simulink model "FRNmodel"  (Simulink 7.9)
settings: Solver=VariableStepDiscrete  StartTime=0.0  StopTime=100.0  RelTol=1e-3
libraries: simeventslib x22, FRN_Library x11
(part 2 of 2)

== system FRNmodel/LTL/Calculate_OUTFlow ==
  Calculate_OUTFlow : MATLAB Function  TreatAsAtomicUnit=on
  Entity Combiner : EntityCombiner  NumberInputPorts=2
  Entity Sink : EntitySink
  Entity Splitter : EntitySplitter  NumberOutputPorts=2
  FIFO Queue : FIFOQueue  Capacity=inf
  Get Attribute : GetAttribute  AttributeName=UoH|Quantity|OUTFlow  AttributeMissing=Error|Error|Error  AttributeDefaultValue=1|1|1  AttributeTreatAsVector=1|1|1  AttributeSendTiming=After entity departure|After entity departure|After entity departure  EvaluatedDefaultAttributeValue={[];[];[]}
      settings: OutputPortMap=o1,o2,o3
  Set Attribute : SetAttribute  AttributeName=OUTFlow  AttributeFrom=Signal port  EvaluatedAttributeValue={[]}
  Single Server : SingleServer  ServiceTime=0
  FlowRecord_IN : PMIOPort  Port=1  Side=Left
  FlowRecord_OUT : PMIOPort  Port=2  Side=Left
  OUTFlow_Signal : PMIOPort  Port=3  Side=Right
  wires:
  Get Attribute/3 -> Calculate_OUTFlow/3(OUTFlow)
  Get Attribute/2 -> Calculate_OUTFlow/2(Quantity)
  Calculate_OUTFlow/1(OUTFlow_return) -> Set Attribute/1
  Get Attribute/1 -> Calculate_OUTFlow/1(UoH)
  connections:
  Entity Splitter/RConn2 -- Entity Sink/LConn1
  FIFO Queue/RConn1 -- Entity Combiner/LConn2
  OUTFlow_Signal/RConn1 -- FIFO Queue/LConn1
  FlowRecord_IN/RConn1 -- Entity Combiner/LConn1
  FlowRecord_OUT/RConn1 -- Entity Splitter/RConn1
  Single Server/RConn1 -- Set Attribute/LConn1
  Get Attribute/RConn1 -- Single Server/LConn1
  Set Attribute/RConn1 -- Entity Splitter/LConn1
  Entity Combiner/RConn1 -- Get Attribute/LConn1

== system FRNmodel/LTL/FlowRecord ==
  FIFO Queue : FIFOQueue
  FlowRecord : TimeBasedFunctionCallGenerator  EventGenerationMode=Only at simulation start
  Get Attribute : GetAttribute  AttributeName=OUTFlow|INFlow  AttributeMissing=Error|Error  AttributeDefaultValue=1|1  AttributeTreatAsVector=1|1  AttributeSendTiming=After entity departure|After entity departure  EvaluatedDefaultAttributeValue={[];[]}
      settings: OutputPortMap=o1,o2
  INFlow_Metric : simeventslib/SimEvents Sinks/Discrete Event Signal to Workspace  VariableName=INFlow_Metric_LTL  SaveFormat=Structure With Time  isMonitorOnly=off  isRecordIC=off
  Initialize_FlowRecord : SetAttribute  AttributeName=INFlow|OUTFlow  AttributeFrom=Dialog|Dialog  AttributeValue=[0 0 0 0 0]|[0 0 0 0 0]  AttributeTreatAsVector=1|1  EvaluatedAttributeValue={[0 0 0 0 0];[0 0 0 0 0]}
  New_FlowRecord : EventBasedEntityGenerator  GenerateEntitiesUpon=Function call from port fcn
  OUTFlow_Metric : simeventslib/SimEvents Sinks/Discrete Event Signal to Workspace  VariableName=OUTFlow_Metric_LTL  SaveFormat=Structure With Time  isMonitorOnly=off  isRecordIC=off
  Output Switch : OutputSwitch  NumberOutputPorts=2
  Path Combiner1 : PathCombiner
  TO_INFlow : PMIOPort  Port=1  Side=Right
  TO_OUTFlow : PMIOPort  Port=2  Side=Left
  FROM_INFlow : PMIOPort  Port=3  Side=Right
  FROM_OUTFlow : PMIOPort  Port=4  Side=Left
  wires:
  Get Attribute/2 -> INFlow_Metric/1
  Get Attribute/1 -> OUTFlow_Metric/1
  FlowRecord/1 -> New_FlowRecord/1
  connections:
  Get Attribute/RConn1 -- FIFO Queue/LConn1
  Path Combiner1/RConn1 -- Get Attribute/LConn1
  FROM_OUTFlow/RConn1 -- Path Combiner1/LConn3
  FROM_INFlow/RConn1 -- Path Combiner1/LConn2
  TO_OUTFlow/RConn1 -- Output Switch/RConn2
  TO_INFlow/RConn1 -- Output Switch/RConn1
  Initialize_FlowRecord/RConn1 -- Path Combiner1/LConn1
  New_FlowRecord/RConn1 -- Initialize_FlowRecord/LConn1
  Output Switch/LConn1 -- FIFO Queue/RConn1

== system FRNmodel/MixedPallet/Calculate_INFlow ==
  Calculate_INFlow : MATLAB Function  TreatAsAtomicUnit=on
  Entity Combiner : EntityCombiner  NumberInputPorts=2
  Entity Sink : EntitySink
  Entity Splitter : EntitySplitter  NumberOutputPorts=2
  FIFO Queue : FIFOQueue  Capacity=inf
  Get Attribute : GetAttribute  AttributeName=UoH|Quantity|INFlow  AttributeMissing=Error|Error|Error  AttributeDefaultValue=1|1|1  AttributeTreatAsVector=1|1|1  AttributeSendTiming=After entity departure|After entity departure|After entity departure  EvaluatedDefaultAttributeValue={[];[];[]}
      settings: OutputPortMap=o1,o2,o3
  Set Attribute : SetAttribute  AttributeName=INFlow  AttributeFrom=Signal port  EvaluatedAttributeValue={[]}
  Single Server : SingleServer  ServiceTime=0
  FlowRecord_IN : PMIOPort  Port=1  Side=Right
  FlowRecord_OUT : PMIOPort  Port=2  Side=Right
  INFlow_Signal : PMIOPort  Port=3  Side=Left
  wires:
  Get Attribute/3 -> Calculate_INFlow/3(INFlow)
  Get Attribute/2 -> Calculate_INFlow/2(Quantity)
  Calculate_INFlow/1(INFlow_return) -> Set Attribute/1
  Get Attribute/1 -> Calculate_INFlow/1(UoH)
  connections:
  FIFO Queue/RConn1 -- Entity Combiner/LConn2
  INFlow_Signal/RConn1 -- FIFO Queue/LConn1
  Entity Splitter/RConn2 -- Entity Sink/LConn1
  FlowRecord_IN/RConn1 -- Entity Combiner/LConn1
  FlowRecord_OUT/RConn1 -- Entity Splitter/RConn1
  Single Server/RConn1 -- Set Attribute/LConn1
  Get Attribute/RConn1 -- Single Server/LConn1
  Set Attribute/RConn1 -- Entity Splitter/LConn1
  Entity Combiner/RConn1 -- Get Attribute/LConn1

== system FRNmodel/MixedPallet/Calculate_OUTFlow ==
  Calculate_OUTFlow : MATLAB Function  TreatAsAtomicUnit=on
  Entity Combiner : EntityCombiner  NumberInputPorts=2
  Entity Sink : EntitySink
  Entity Splitter : EntitySplitter  NumberOutputPorts=2
  FIFO Queue : FIFOQueue  Capacity=inf
  Get Attribute : GetAttribute  AttributeName=UoH|Quantity|OUTFlow  AttributeMissing=Error|Error|Error  AttributeDefaultValue=1|1|1  AttributeTreatAsVector=1|1|1  AttributeSendTiming=After entity departure|After entity departure|After entity departure  EvaluatedDefaultAttributeValue={[];[];[]}
      settings: OutputPortMap=o1,o2,o3
  Set Attribute : SetAttribute  AttributeName=OUTFlow  AttributeFrom=Signal port  EvaluatedAttributeValue={[]}
  Single Server : SingleServer  ServiceTime=0
  FlowRecord_IN : PMIOPort  Port=1  Side=Left
  FlowRecord_OUT : PMIOPort  Port=2  Side=Left
  OUTFlow_Signal : PMIOPort  Port=3  Side=Right
  wires:
  Get Attribute/3 -> Calculate_OUTFlow/3(OUTFlow)
  Get Attribute/2 -> Calculate_OUTFlow/2(Quantity)
  Calculate_OUTFlow/1(OUTFlow_return) -> Set Attribute/1
  Get Attribute/1 -> Calculate_OUTFlow/1(UoH)
  connections:
  Entity Splitter/RConn2 -- Entity Sink/LConn1
  FIFO Queue/RConn1 -- Entity Combiner/LConn2
  OUTFlow_Signal/RConn1 -- FIFO Queue/LConn1
  FlowRecord_IN/RConn1 -- Entity Combiner/LConn1
  FlowRecord_OUT/RConn1 -- Entity Splitter/RConn1
  Single Server/RConn1 -- Set Attribute/LConn1
  Get Attribute/RConn1 -- Single Server/LConn1
  Set Attribute/RConn1 -- Entity Splitter/LConn1
  Entity Combiner/RConn1 -- Get Attribute/LConn1

== system FRNmodel/MixedPallet/FlowRecord ==
  FIFO Queue : FIFOQueue
  FlowRecord : TimeBasedFunctionCallGenerator  EventGenerationMode=Only at simulation start
  Get Attribute : GetAttribute  AttributeName=OUTFlow|INFlow  AttributeMissing=Error|Error  AttributeDefaultValue=1|1  AttributeTreatAsVector=1|1  AttributeSendTiming=After entity departure|After entity departure  EvaluatedDefaultAttributeValue={[];[]}
      settings: OutputPortMap=o1,o2
  INFlow_Metric : simeventslib/SimEvents Sinks/Discrete Event Signal to Workspace  VariableName=INFlow_Metric_MixedPallet  SaveFormat=Structure With Time  isMonitorOnly=off  isRecordIC=off
  Initialize_FlowRecord : SetAttribute  AttributeName=INFlow|OUTFlow  AttributeFrom=Dialog|Dialog  AttributeValue=[0 0 0 0 0]|[0 0 0 0 0]  AttributeTreatAsVector=1|1  EvaluatedAttributeValue={[0 0 0 0 0];[0 0 0 0 0]}
  New_FlowRecord : EventBasedEntityGenerator  GenerateEntitiesUpon=Function call from port fcn
  OUTFlow_Metric : simeventslib/SimEvents Sinks/Discrete Event Signal to Workspace  VariableName=OUTFlow_Metric_MixedPallet  SaveFormat=Structure With Time  isMonitorOnly=off  isRecordIC=off
  Output Switch : OutputSwitch  NumberOutputPorts=2
  Path Combiner1 : PathCombiner
  TO_INFlow : PMIOPort  Port=1  Side=Right
  TO_OUTFlow : PMIOPort  Port=2  Side=Left
  FROM_INFlow : PMIOPort  Port=3  Side=Right
  FROM_OUTFlow : PMIOPort  Port=4  Side=Left
  wires:
  Get Attribute/2 -> INFlow_Metric/1
  Get Attribute/1 -> OUTFlow_Metric/1
  FlowRecord/1 -> New_FlowRecord/1
  connections:
  Get Attribute/RConn1 -- FIFO Queue/LConn1
  Path Combiner1/RConn1 -- Get Attribute/LConn1
  FROM_OUTFlow/RConn1 -- Path Combiner1/LConn3
  FROM_INFlow/RConn1 -- Path Combiner1/LConn2
  TO_OUTFlow/RConn1 -- Output Switch/RConn2
  TO_INFlow/RConn1 -- Output Switch/RConn1
  Initialize_FlowRecord/RConn1 -- Path Combiner1/LConn1
  New_FlowRecord/RConn1 -- Initialize_FlowRecord/LConn1
  Output Switch/LConn1 -- FIFO Queue/RConn1

== system FRNmodel/PickFastCarton/Calculate_INFlow ==
  Calculate_INFlow : MATLAB Function  TreatAsAtomicUnit=on
  Entity Combiner : EntityCombiner  NumberInputPorts=2
  Entity Sink : EntitySink
  Entity Splitter : EntitySplitter  NumberOutputPorts=2
  FIFO Queue : FIFOQueue  Capacity=inf
  Get Attribute : GetAttribute  AttributeName=UoH|Quantity|INFlow  AttributeMissing=Error|Error|Error  AttributeDefaultValue=1|1|1  AttributeTreatAsVector=1|1|1  AttributeSendTiming=After entity departure|After entity departure|After entity departure  EvaluatedDefaultAttributeValue={[];[];[]}
      settings: OutputPortMap=o1,o2,o3
  Set Attribute : SetAttribute  AttributeName=INFlow  AttributeFrom=Signal port  EvaluatedAttributeValue={[]}
  Single Server : SingleServer  ServiceTime=0
  FlowRecord_IN : PMIOPort  Port=1  Side=Right
  FlowRecord_OUT : PMIOPort  Port=2  Side=Right
  INFlow_Signal : PMIOPort  Port=3  Side=Left
  wires:
  Get Attribute/3 -> Calculate_INFlow/3(INFlow)
  Get Attribute/2 -> Calculate_INFlow/2(Quantity)
  Calculate_INFlow/1(INFlow_return) -> Set Attribute/1
  Get Attribute/1 -> Calculate_INFlow/1(UoH)
  connections:
  FIFO Queue/RConn1 -- Entity Combiner/LConn2
  INFlow_Signal/RConn1 -- FIFO Queue/LConn1
  Entity Splitter/RConn2 -- Entity Sink/LConn1
  FlowRecord_IN/RConn1 -- Entity Combiner/LConn1
  FlowRecord_OUT/RConn1 -- Entity Splitter/RConn1
  Single Server/RConn1 -- Set Attribute/LConn1
  Get Attribute/RConn1 -- Single Server/LConn1
  Set Attribute/RConn1 -- Entity Splitter/LConn1
  Entity Combiner/RConn1 -- Get Attribute/LConn1

== system FRNmodel/PickFastCarton/Calculate_OUTFlow ==
  Calculate_OUTFlow : MATLAB Function  TreatAsAtomicUnit=on
  Entity Combiner : EntityCombiner  NumberInputPorts=2
  Entity Sink : EntitySink
  Entity Splitter : EntitySplitter  NumberOutputPorts=2
  FIFO Queue : FIFOQueue  Capacity=inf
  Get Attribute : GetAttribute  AttributeName=UoH|Quantity|OUTFlow  AttributeMissing=Error|Error|Error  AttributeDefaultValue=1|1|1  AttributeTreatAsVector=1|1|1  AttributeSendTiming=After entity departure|After entity departure|After entity departure  EvaluatedDefaultAttributeValue={[];[];[]}
      settings: OutputPortMap=o1,o2,o3
  Set Attribute : SetAttribute  AttributeName=OUTFlow  AttributeFrom=Signal port  EvaluatedAttributeValue={[]}
  Single Server : SingleServer  ServiceTime=0
  FlowRecord_IN : PMIOPort  Port=1  Side=Left
  FlowRecord_OUT : PMIOPort  Port=2  Side=Left
  OUTFlow_Signal : PMIOPort  Port=3  Side=Right
  wires:
  Get Attribute/3 -> Calculate_OUTFlow/3(OUTFlow)
  Get Attribute/2 -> Calculate_OUTFlow/2(Quantity)
  Calculate_OUTFlow/1(OUTFlow_return) -> Set Attribute/1
  Get Attribute/1 -> Calculate_OUTFlow/1(UoH)
  connections:
  Entity Splitter/RConn2 -- Entity Sink/LConn1
  FIFO Queue/RConn1 -- Entity Combiner/LConn2
  OUTFlow_Signal/RConn1 -- FIFO Queue/LConn1
  FlowRecord_IN/RConn1 -- Entity Combiner/LConn1
  FlowRecord_OUT/RConn1 -- Entity Splitter/RConn1
  Single Server/RConn1 -- Set Attribute/LConn1
  Get Attribute/RConn1 -- Single Server/LConn1
  Set Attribute/RConn1 -- Entity Splitter/LConn1
  Entity Combiner/RConn1 -- Get Attribute/LConn1

== system FRNmodel/PickFastCarton/FlowRecord ==
  FIFO Queue : FIFOQueue
  FlowRecord : TimeBasedFunctionCallGenerator  EventGenerationMode=Only at simulation start
  Get Attribute : GetAttribute  AttributeName=OUTFlow|INFlow  AttributeMissing=Error|Error  AttributeDefaultValue=1|1  AttributeTreatAsVector=1|1  AttributeSendTiming=After entity departure|After entity departure  EvaluatedDefaultAttributeValue={[];[]}
      settings: OutputPortMap=o1,o2
  INFlow_Metric : simeventslib/SimEvents Sinks/Discrete Event Signal to Workspace  VariableName=INFlow_Metric_PickFastCarton  SaveFormat=Structure With Time  isMonitorOnly=off  isRecordIC=off
  Initialize_FlowRecord : SetAttribute  AttributeName=INFlow|OUTFlow  AttributeFrom=Dialog|Dialog  AttributeValue=[0 0 0 0 0]|[0 0 0 0 0]  AttributeTreatAsVector=1|1  EvaluatedAttributeValue={[0 0 0 0 0];[0 0 0 0 0]}
  New_FlowRecord : EventBasedEntityGenerator  GenerateEntitiesUpon=Function call from port fcn
  OUTFlow_Metric : simeventslib/SimEvents Sinks/Discrete Event Signal to Workspace  VariableName=OUTFlow_Metric_PickFastCarton  SaveFormat=Structure With Time  isMonitorOnly=off  isRecordIC=off
  Output Switch : OutputSwitch  NumberOutputPorts=2
  Path Combiner1 : PathCombiner
  TO_INFlow : PMIOPort  Port=1  Side=Right
  TO_OUTFlow : PMIOPort  Port=2  Side=Left
  FROM_INFlow : PMIOPort  Port=3  Side=Right
  FROM_OUTFlow : PMIOPort  Port=4  Side=Left
  wires:
  Get Attribute/2 -> INFlow_Metric/1
  Get Attribute/1 -> OUTFlow_Metric/1
  FlowRecord/1 -> New_FlowRecord/1
  connections:
  Get Attribute/RConn1 -- FIFO Queue/LConn1
  Path Combiner1/RConn1 -- Get Attribute/LConn1
  FROM_OUTFlow/RConn1 -- Path Combiner1/LConn3
  FROM_INFlow/RConn1 -- Path Combiner1/LConn2
  TO_OUTFlow/RConn1 -- Output Switch/RConn2
  TO_INFlow/RConn1 -- Output Switch/RConn1
  Initialize_FlowRecord/RConn1 -- Path Combiner1/LConn1
  New_FlowRecord/RConn1 -- Initialize_FlowRecord/LConn1
  Output Switch/LConn1 -- FIFO Queue/RConn1

== system FRNmodel/PickHeavyCarton/Calculate_INFlow ==
  Calculate_INFlow : MATLAB Function  TreatAsAtomicUnit=on
  Entity Combiner : EntityCombiner  NumberInputPorts=2
  Entity Sink : EntitySink
  Entity Splitter : EntitySplitter  NumberOutputPorts=2
  FIFO Queue : FIFOQueue  Capacity=inf
  Get Attribute : GetAttribute  AttributeName=UoH|Quantity|INFlow  AttributeMissing=Error|Error|Error  AttributeDefaultValue=1|1|1  AttributeTreatAsVector=1|1|1  AttributeSendTiming=After entity departure|After entity departure|After entity departure  EvaluatedDefaultAttributeValue={[];[];[]}
      settings: OutputPortMap=o1,o2,o3
  Set Attribute : SetAttribute  AttributeName=INFlow  AttributeFrom=Signal port  EvaluatedAttributeValue={[]}
  Single Server : SingleServer  ServiceTime=0
  FlowRecord_IN : PMIOPort  Port=1  Side=Right
  FlowRecord_OUT : PMIOPort  Port=2  Side=Right
  INFlow_Signal : PMIOPort  Port=3  Side=Left
  wires:
  Get Attribute/3 -> Calculate_INFlow/3(INFlow)
  Get Attribute/2 -> Calculate_INFlow/2(Quantity)
  Calculate_INFlow/1(INFlow_return) -> Set Attribute/1
  Get Attribute/1 -> Calculate_INFlow/1(UoH)
  connections:
  FIFO Queue/RConn1 -- Entity Combiner/LConn2
  INFlow_Signal/RConn1 -- FIFO Queue/LConn1
  Entity Splitter/RConn2 -- Entity Sink/LConn1
  FlowRecord_IN/RConn1 -- Entity Combiner/LConn1
  FlowRecord_OUT/RConn1 -- Entity Splitter/RConn1
  Single Server/RConn1 -- Set Attribute/LConn1
  Get Attribute/RConn1 -- Single Server/LConn1
  Set Attribute/RConn1 -- Entity Splitter/LConn1
  Entity Combiner/RConn1 -- Get Attribute/LConn1

== system FRNmodel/PickHeavyCarton/Calculate_OUTFlow ==
  Calculate_OUTFlow : MATLAB Function  TreatAsAtomicUnit=on
  Entity Combiner : EntityCombiner  NumberInputPorts=2
  Entity Sink : EntitySink
  Entity Splitter : EntitySplitter  NumberOutputPorts=2
  FIFO Queue : FIFOQueue  Capacity=inf
  Get Attribute : GetAttribute  AttributeName=UoH|Quantity|OUTFlow  AttributeMissing=Error|Error|Error  AttributeDefaultValue=1|1|1  AttributeTreatAsVector=1|1|1  AttributeSendTiming=After entity departure|After entity departure|After entity departure  EvaluatedDefaultAttributeValue={[];[];[]}
      settings: OutputPortMap=o1,o2,o3
  Set Attribute : SetAttribute  AttributeName=OUTFlow  AttributeFrom=Signal port  EvaluatedAttributeValue={[]}
  Single Server : SingleServer  ServiceTime=0
  FlowRecord_IN : PMIOPort  Port=1  Side=Left
  FlowRecord_OUT : PMIOPort  Port=2  Side=Left
  OUTFlow_Signal : PMIOPort  Port=3  Side=Right
  wires:
  Get Attribute/3 -> Calculate_OUTFlow/3(OUTFlow)
  Get Attribute/2 -> Calculate_OUTFlow/2(Quantity)
  Calculate_OUTFlow/1(OUTFlow_return) -> Set Attribute/1
  Get Attribute/1 -> Calculate_OUTFlow/1(UoH)
  connections:
  Entity Splitter/RConn2 -- Entity Sink/LConn1
  FIFO Queue/RConn1 -- Entity Combiner/LConn2
  OUTFlow_Signal/RConn1 -- FIFO Queue/LConn1
  FlowRecord_IN/RConn1 -- Entity Combiner/LConn1
  FlowRecord_OUT/RConn1 -- Entity Splitter/RConn1
  Single Server/RConn1 -- Set Attribute/LConn1
  Get Attribute/RConn1 -- Single Server/LConn1
  Set Attribute/RConn1 -- Entity Splitter/LConn1
  Entity Combiner/RConn1 -- Get Attribute/LConn1

== system FRNmodel/PickHeavyCarton/FlowRecord ==
  FIFO Queue : FIFOQueue
  FlowRecord : TimeBasedFunctionCallGenerator  EventGenerationMode=Only at simulation start
  Get Attribute : GetAttribute  AttributeName=OUTFlow|INFlow  AttributeMissing=Error|Error  AttributeDefaultValue=1|1  AttributeTreatAsVector=1|1  AttributeSendTiming=After entity departure|After entity departure  EvaluatedDefaultAttributeValue={[];[]}
      settings: OutputPortMap=o1,o2
  INFlow_Metric : simeventslib/SimEvents Sinks/Discrete Event Signal to Workspace  VariableName=INFlow_Metric_PickHeavyCarton  SaveFormat=Structure With Time  isMonitorOnly=off  isRecordIC=off
  Initialize_FlowRecord : SetAttribute  AttributeName=INFlow|OUTFlow  AttributeFrom=Dialog|Dialog  AttributeValue=[0 0 0 0 0]|[0 0 0 0 0]  AttributeTreatAsVector=1|1  EvaluatedAttributeValue={[0 0 0 0 0];[0 0 0 0 0]}
  New_FlowRecord : EventBasedEntityGenerator  GenerateEntitiesUpon=Function call from port fcn
  OUTFlow_Metric : simeventslib/SimEvents Sinks/Discrete Event Signal to Workspace  VariableName=OUTFlow_Metric_PickHeavyCarton  SaveFormat=Structure With Time  isMonitorOnly=off  isRecordIC=off
  Output Switch : OutputSwitch  NumberOutputPorts=2
  Path Combiner1 : PathCombiner
  TO_INFlow : PMIOPort  Port=1  Side=Right
  TO_OUTFlow : PMIOPort  Port=2  Side=Left
  FROM_INFlow : PMIOPort  Port=3  Side=Right
  FROM_OUTFlow : PMIOPort  Port=4  Side=Left
  wires:
  Get Attribute/2 -> INFlow_Metric/1
  Get Attribute/1 -> OUTFlow_Metric/1
  FlowRecord/1 -> New_FlowRecord/1
  connections:
  Get Attribute/RConn1 -- FIFO Queue/LConn1
  Path Combiner1/RConn1 -- Get Attribute/LConn1
  FROM_OUTFlow/RConn1 -- Path Combiner1/LConn3
  FROM_INFlow/RConn1 -- Path Combiner1/LConn2
  TO_OUTFlow/RConn1 -- Output Switch/RConn2
  TO_INFlow/RConn1 -- Output Switch/RConn1
  Initialize_FlowRecord/RConn1 -- Path Combiner1/LConn1
  New_FlowRecord/RConn1 -- Initialize_FlowRecord/LConn1
  Output Switch/LConn1 -- FIFO Queue/RConn1

== system FRNmodel/PickSlowCarton/Calculate_INFlow ==
  Calculate_INFlow : MATLAB Function  TreatAsAtomicUnit=on
  Entity Combiner : EntityCombiner  NumberInputPorts=2
  Entity Sink : EntitySink
  Entity Splitter : EntitySplitter  NumberOutputPorts=2
  FIFO Queue : FIFOQueue  Capacity=inf
  Get Attribute : GetAttribute  AttributeName=UoH|Quantity|INFlow  AttributeMissing=Error|Error|Error  AttributeDefaultValue=1|1|1  AttributeTreatAsVector=1|1|1  AttributeSendTiming=After entity departure|After entity departure|After entity departure  EvaluatedDefaultAttributeValue={[];[];[]}
      settings: OutputPortMap=o1,o2,o3
  Set Attribute : SetAttribute  AttributeName=INFlow  AttributeFrom=Signal port  EvaluatedAttributeValue={[]}
  Single Server : SingleServer  ServiceTime=0
  FlowRecord_IN : PMIOPort  Port=1  Side=Right
  FlowRecord_OUT : PMIOPort  Port=2  Side=Right
  INFlow_Signal : PMIOPort  Port=3  Side=Left
  wires:
  Get Attribute/3 -> Calculate_INFlow/3(INFlow)
  Get Attribute/2 -> Calculate_INFlow/2(Quantity)
  Calculate_INFlow/1(INFlow_return) -> Set Attribute/1
  Get Attribute/1 -> Calculate_INFlow/1(UoH)
  connections:
  FIFO Queue/RConn1 -- Entity Combiner/LConn2
  INFlow_Signal/RConn1 -- FIFO Queue/LConn1
  Entity Splitter/RConn2 -- Entity Sink/LConn1
  FlowRecord_IN/RConn1 -- Entity Combiner/LConn1
  FlowRecord_OUT/RConn1 -- Entity Splitter/RConn1
  Single Server/RConn1 -- Set Attribute/LConn1
  Get Attribute/RConn1 -- Single Server/LConn1
  Set Attribute/RConn1 -- Entity Splitter/LConn1
  Entity Combiner/RConn1 -- Get Attribute/LConn1

== system FRNmodel/PickSlowCarton/Calculate_OUTFlow ==
  Calculate_OUTFlow : MATLAB Function  TreatAsAtomicUnit=on
  Entity Combiner : EntityCombiner  NumberInputPorts=2
  Entity Sink : EntitySink
  Entity Splitter : EntitySplitter  NumberOutputPorts=2
  FIFO Queue : FIFOQueue  Capacity=inf
  Get Attribute : GetAttribute  AttributeName=UoH|Quantity|OUTFlow  AttributeMissing=Error|Error|Error  AttributeDefaultValue=1|1|1  AttributeTreatAsVector=1|1|1  AttributeSendTiming=After entity departure|After entity departure|After entity departure  EvaluatedDefaultAttributeValue={[];[];[]}
      settings: OutputPortMap=o1,o2,o3
  Set Attribute : SetAttribute  AttributeName=OUTFlow  AttributeFrom=Signal port  EvaluatedAttributeValue={[]}
  Single Server : SingleServer  ServiceTime=0
  FlowRecord_IN : PMIOPort  Port=1  Side=Left
  FlowRecord_OUT : PMIOPort  Port=2  Side=Left
  OUTFlow_Signal : PMIOPort  Port=3  Side=Right
  wires:
  Get Attribute/3 -> Calculate_OUTFlow/3(OUTFlow)
  Get Attribute/2 -> Calculate_OUTFlow/2(Quantity)
  Calculate_OUTFlow/1(OUTFlow_return) -> Set Attribute/1
  Get Attribute/1 -> Calculate_OUTFlow/1(UoH)
  connections:
  Entity Splitter/RConn2 -- Entity Sink/LConn1
  FIFO Queue/RConn1 -- Entity Combiner/LConn2
  OUTFlow_Signal/RConn1 -- FIFO Queue/LConn1
  FlowRecord_IN/RConn1 -- Entity Combiner/LConn1
  FlowRecord_OUT/RConn1 -- Entity Splitter/RConn1
  Single Server/RConn1 -- Set Attribute/LConn1
  Get Attribute/RConn1 -- Single Server/LConn1
  Set Attribute/RConn1 -- Entity Splitter/LConn1
  Entity Combiner/RConn1 -- Get Attribute/LConn1

== system FRNmodel/PickSlowCarton/FlowRecord ==
  FIFO Queue : FIFOQueue
  FlowRecord : TimeBasedFunctionCallGenerator  EventGenerationMode=Only at simulation start
  Get Attribute : GetAttribute  AttributeName=OUTFlow|INFlow  AttributeMissing=Error|Error  AttributeDefaultValue=1|1  AttributeTreatAsVector=1|1  AttributeSendTiming=After entity departure|After entity departure  EvaluatedDefaultAttributeValue={[];[]}
      settings: OutputPortMap=o1,o2
  INFlow_Metric : simeventslib/SimEvents Sinks/Discrete Event Signal to Workspace  VariableName=INFlow_Metric_PickSlowCarton  SaveFormat=Structure With Time  isMonitorOnly=off  isRecordIC=off
  Initialize_FlowRecord : SetAttribute  AttributeName=INFlow|OUTFlow  AttributeFrom=Dialog|Dialog  AttributeValue=[0 0 0 0 0]|[0 0 0 0 0]  AttributeTreatAsVector=1|1  EvaluatedAttributeValue={[0 0 0 0 0];[0 0 0 0 0]}
  New_FlowRecord : EventBasedEntityGenerator  GenerateEntitiesUpon=Function call from port fcn
  OUTFlow_Metric : simeventslib/SimEvents Sinks/Discrete Event Signal to Workspace  VariableName=OUTFlow_Metric_PickSlowCarton  SaveFormat=Structure With Time  isMonitorOnly=off  isRecordIC=off
  Output Switch : OutputSwitch  NumberOutputPorts=2
  Path Combiner1 : PathCombiner
  TO_INFlow : PMIOPort  Port=1  Side=Right
  TO_OUTFlow : PMIOPort  Port=2  Side=Left
  FROM_INFlow : PMIOPort  Port=3  Side=Right
  FROM_OUTFlow : PMIOPort  Port=4  Side=Left
  wires:
  Get Attribute/2 -> INFlow_Metric/1
  Get Attribute/1 -> OUTFlow_Metric/1
  FlowRecord/1 -> New_FlowRecord/1
  connections:
  Get Attribute/RConn1 -- FIFO Queue/LConn1
  Path Combiner1/RConn1 -- Get Attribute/LConn1
  FROM_OUTFlow/RConn1 -- Path Combiner1/LConn3
  FROM_INFlow/RConn1 -- Path Combiner1/LConn2
  TO_OUTFlow/RConn1 -- Output Switch/RConn2
  TO_INFlow/RConn1 -- Output Switch/RConn1
  Initialize_FlowRecord/RConn1 -- Path Combiner1/LConn1
  New_FlowRecord/RConn1 -- Initialize_FlowRecord/LConn1
  Output Switch/LConn1 -- FIFO Queue/RConn1

== system FRNmodel/SlowCarton2MPassembly/Calculate_INFlow ==
  Calculate_INFlow : MATLAB Function  TreatAsAtomicUnit=on
  Entity Combiner : EntityCombiner  NumberInputPorts=2
  Entity Sink : EntitySink
  Entity Splitter : EntitySplitter  NumberOutputPorts=2
  FIFO Queue : FIFOQueue  Capacity=inf
  Get Attribute : GetAttribute  AttributeName=UoH|Quantity|INFlow  AttributeMissing=Error|Error|Error  AttributeDefaultValue=1|1|1  AttributeTreatAsVector=1|1|1  AttributeSendTiming=After entity departure|After entity departure|After entity departure  EvaluatedDefaultAttributeValue={[];[];[]}
      settings: OutputPortMap=o1,o2,o3
  Set Attribute : SetAttribute  AttributeName=INFlow  AttributeFrom=Signal port  EvaluatedAttributeValue={[]}
  Single Server : SingleServer  ServiceTime=0
  FlowRecord_IN : PMIOPort  Port=1  Side=Right
  FlowRecord_OUT : PMIOPort  Port=2  Side=Right
  INFlow_Signal : PMIOPort  Port=3  Side=Left
  wires:
  Get Attribute/3 -> Calculate_INFlow/3(INFlow)
  Get Attribute/2 -> Calculate_INFlow/2(Quantity)
  Calculate_INFlow/1(INFlow_return) -> Set Attribute/1
  Get Attribute/1 -> Calculate_INFlow/1(UoH)
  connections:
  FIFO Queue/RConn1 -- Entity Combiner/LConn2
  INFlow_Signal/RConn1 -- FIFO Queue/LConn1
  Entity Splitter/RConn2 -- Entity Sink/LConn1
  FlowRecord_IN/RConn1 -- Entity Combiner/LConn1
  FlowRecord_OUT/RConn1 -- Entity Splitter/RConn1
  Single Server/RConn1 -- Set Attribute/LConn1
  Get Attribute/RConn1 -- Single Server/LConn1
  Set Attribute/RConn1 -- Entity Splitter/LConn1
  Entity Combiner/RConn1 -- Get Attribute/LConn1

== system FRNmodel/SlowCarton2MPassembly/Calculate_OUTFlow ==
  Calculate_OUTFlow : MATLAB Function  TreatAsAtomicUnit=on
  Entity Combiner : EntityCombiner  NumberInputPorts=2
  Entity Sink : EntitySink
  Entity Splitter : EntitySplitter  NumberOutputPorts=2
  FIFO Queue : FIFOQueue  Capacity=inf
  Get Attribute : GetAttribute  AttributeName=UoH|Quantity|OUTFlow  AttributeMissing=Error|Error|Error  AttributeDefaultValue=1|1|1  AttributeTreatAsVector=1|1|1  AttributeSendTiming=After entity departure|After entity departure|After entity departure  EvaluatedDefaultAttributeValue={[];[];[]}
      settings: OutputPortMap=o1,o2,o3
  Set Attribute : SetAttribute  AttributeName=OUTFlow  AttributeFrom=Signal port  EvaluatedAttributeValue={[]}
  Single Server : SingleServer  ServiceTime=0
  FlowRecord_IN : PMIOPort  Port=1  Side=Left
  FlowRecord_OUT : PMIOPort  Port=2  Side=Left
  OUTFlow_Signal : PMIOPort  Port=3  Side=Right
  wires:
  Get Attribute/3 -> Calculate_OUTFlow/3(OUTFlow)
  Get Attribute/2 -> Calculate_OUTFlow/2(Quantity)
  Calculate_OUTFlow/1(OUTFlow_return) -> Set Attribute/1
  Get Attribute/1 -> Calculate_OUTFlow/1(UoH)
  connections:
  Entity Splitter/RConn2 -- Entity Sink/LConn1
  FIFO Queue/RConn1 -- Entity Combiner/LConn2
  OUTFlow_Signal/RConn1 -- FIFO Queue/LConn1
  FlowRecord_IN/RConn1 -- Entity Combiner/LConn1
  FlowRecord_OUT/RConn1 -- Entity Splitter/RConn1
  Single Server/RConn1 -- Set Attribute/LConn1
  Get Attribute/RConn1 -- Single Server/LConn1
  Set Attribute/RConn1 -- Entity Splitter/LConn1
  Entity Combiner/RConn1 -- Get Attribute/LConn1

== system FRNmodel/SlowCarton2MPassembly/FlowRecord ==
  FIFO Queue : FIFOQueue
  FlowRecord : TimeBasedFunctionCallGenerator  EventGenerationMode=Only at simulation start
  Get Attribute : GetAttribute  AttributeName=OUTFlow|INFlow  AttributeMissing=Error|Error  AttributeDefaultValue=1|1  AttributeTreatAsVector=1|1  AttributeSendTiming=After entity departure|After entity departure  EvaluatedDefaultAttributeValue={[];[]}
      settings: OutputPortMap=o1,o2
  INFlow_Metric : simeventslib/SimEvents Sinks/Discrete Event Signal to Workspace  VariableName=INFlow_Metric_SlowCarton2MPassembly  SaveFormat=Structure With Time  isMonitorOnly=off  isRecordIC=off
  Initialize_FlowRecord : SetAttribute  AttributeName=INFlow|OUTFlow  AttributeFrom=Dialog|Dialog  AttributeValue=[0 0 0 0 0]|[0 0 0 0 0]  AttributeTreatAsVector=1|1  EvaluatedAttributeValue={[0 0 0 0 0];[0 0 0 0 0]}
  New_FlowRecord : EventBasedEntityGenerator  GenerateEntitiesUpon=Function call from port fcn
  OUTFlow_Metric : simeventslib/SimEvents Sinks/Discrete Event Signal to Workspace  VariableName=OUTFlow_Metric_SlowCarton2MPassembly  SaveFormat=Structure With Time  isMonitorOnly=off  isRecordIC=off
  Output Switch : OutputSwitch  NumberOutputPorts=2
  Path Combiner1 : PathCombiner
  TO_INFlow : PMIOPort  Port=1  Side=Right
  TO_OUTFlow : PMIOPort  Port=2  Side=Left
  FROM_INFlow : PMIOPort  Port=3  Side=Right
  FROM_OUTFlow : PMIOPort  Port=4  Side=Left
  wires:
  Get Attribute/2 -> INFlow_Metric/1
  Get Attribute/1 -> OUTFlow_Metric/1
  FlowRecord/1 -> New_FlowRecord/1
  connections:
  Get Attribute/RConn1 -- FIFO Queue/LConn1
  Path Combiner1/RConn1 -- Get Attribute/LConn1
  FROM_OUTFlow/RConn1 -- Path Combiner1/LConn3
  FROM_INFlow/RConn1 -- Path Combiner1/LConn2
  TO_OUTFlow/RConn1 -- Output Switch/RConn2
  TO_INFlow/RConn1 -- Output Switch/RConn1
  Initialize_FlowRecord/RConn1 -- Path Combiner1/LConn1
  New_FlowRecord/RConn1 -- Initialize_FlowRecord/LConn1
  Output Switch/LConn1 -- FIFO Queue/RConn1

== system FRNmodel/SlowCartonSTORE/Calculate_INFlow ==
  Calculate_INFlow : MATLAB Function  TreatAsAtomicUnit=on
  Entity Combiner : EntityCombiner  NumberInputPorts=2
  Entity Sink : EntitySink
  Entity Splitter : EntitySplitter  NumberOutputPorts=2
  FIFO Queue : FIFOQueue  Capacity=inf
  Get Attribute : GetAttribute  AttributeName=UoH|Quantity|INFlow  AttributeMissing=Error|Error|Error  AttributeDefaultValue=1|1|1  AttributeTreatAsVector=1|1|1  AttributeSendTiming=After entity departure|After entity departure|After entity departure  EvaluatedDefaultAttributeValue={[];[];[]}
      settings: OutputPortMap=o1,o2,o3
  Set Attribute : SetAttribute  AttributeName=INFlow  AttributeFrom=Signal port  EvaluatedAttributeValue={[]}
  Single Server : SingleServer  ServiceTime=0
  FlowRecord_IN : PMIOPort  Port=1  Side=Right
  FlowRecord_OUT : PMIOPort  Port=2  Side=Right
  INFlow_Signal : PMIOPort  Port=3  Side=Left
  wires:
  Get Attribute/3 -> Calculate_INFlow/3(INFlow)
  Get Attribute/2 -> Calculate_INFlow/2(Quantity)
  Calculate_INFlow/1(INFlow_return) -> Set Attribute/1
  Get Attribute/1 -> Calculate_INFlow/1(UoH)
  connections:
  FIFO Queue/RConn1 -- Entity Combiner/LConn2
  INFlow_Signal/RConn1 -- FIFO Queue/LConn1
  Entity Splitter/RConn2 -- Entity Sink/LConn1
  FlowRecord_IN/RConn1 -- Entity Combiner/LConn1
  FlowRecord_OUT/RConn1 -- Entity Splitter/RConn1
  Single Server/RConn1 -- Set Attribute/LConn1
  Get Attribute/RConn1 -- Single Server/LConn1
  Set Attribute/RConn1 -- Entity Splitter/LConn1
  Entity Combiner/RConn1 -- Get Attribute/LConn1

== system FRNmodel/SlowCartonSTORE/Calculate_OUTFlow ==
  Calculate_OUTFlow : MATLAB Function  TreatAsAtomicUnit=on
  Entity Combiner : EntityCombiner  NumberInputPorts=2
  Entity Sink : EntitySink
  Entity Splitter : EntitySplitter  NumberOutputPorts=2
  FIFO Queue : FIFOQueue  Capacity=inf
  Get Attribute : GetAttribute  AttributeName=UoH|Quantity|OUTFlow  AttributeMissing=Error|Error|Error  AttributeDefaultValue=1|1|1  AttributeTreatAsVector=1|1|1  AttributeSendTiming=After entity departure|After entity departure|After entity departure  EvaluatedDefaultAttributeValue={[];[];[]}
      settings: OutputPortMap=o1,o2,o3
  Set Attribute : SetAttribute  AttributeName=OUTFlow  AttributeFrom=Signal port  EvaluatedAttributeValue={[]}
  Single Server : SingleServer  ServiceTime=0
  FlowRecord_IN : PMIOPort  Port=1  Side=Left
  FlowRecord_OUT : PMIOPort  Port=2  Side=Left
  OUTFlow_Signal : PMIOPort  Port=3  Side=Right
  wires:
  Get Attribute/3 -> Calculate_OUTFlow/3(OUTFlow)
  Get Attribute/2 -> Calculate_OUTFlow/2(Quantity)
  Calculate_OUTFlow/1(OUTFlow_return) -> Set Attribute/1
  Get Attribute/1 -> Calculate_OUTFlow/1(UoH)
  connections:
  Entity Splitter/RConn2 -- Entity Sink/LConn1
  FIFO Queue/RConn1 -- Entity Combiner/LConn2
  OUTFlow_Signal/RConn1 -- FIFO Queue/LConn1
  FlowRecord_IN/RConn1 -- Entity Combiner/LConn1
  FlowRecord_OUT/RConn1 -- Entity Splitter/RConn1
  Single Server/RConn1 -- Set Attribute/LConn1
  Get Attribute/RConn1 -- Single Server/LConn1
  Set Attribute/RConn1 -- Entity Splitter/LConn1
  Entity Combiner/RConn1 -- Get Attribute/LConn1

== system FRNmodel/SlowCartonSTORE/FlowRecord ==
  FIFO Queue : FIFOQueue
  FlowRecord : TimeBasedFunctionCallGenerator  EventGenerationMode=Only at simulation start
  Get Attribute : GetAttribute  AttributeName=OUTFlow|INFlow  AttributeMissing=Error|Error  AttributeDefaultValue=1|1  AttributeTreatAsVector=1|1  AttributeSendTiming=After entity departure|After entity departure  EvaluatedDefaultAttributeValue={[];[]}
      settings: OutputPortMap=o1,o2
  INFlow_Metric : simeventslib/SimEvents Sinks/Discrete Event Signal to Workspace  VariableName=INFlow_Metric_SlowCartonSTORE  SaveFormat=Structure With Time  isMonitorOnly=off  isRecordIC=off
  Initialize_FlowRecord : SetAttribute  AttributeName=INFlow|OUTFlow  AttributeFrom=Dialog|Dialog  AttributeValue=[0 0 0 0 0]|[0 0 0 0 0]  AttributeTreatAsVector=1|1  EvaluatedAttributeValue={[0 0 0 0 0];[0 0 0 0 0]}
  New_FlowRecord : EventBasedEntityGenerator  GenerateEntitiesUpon=Function call from port fcn
  OUTFlow_Metric : simeventslib/SimEvents Sinks/Discrete Event Signal to Workspace  VariableName=OUTFlow_Metric_SlowCartonSTORE  SaveFormat=Structure With Time  isMonitorOnly=off  isRecordIC=off
  Output Switch : OutputSwitch  NumberOutputPorts=2
  Path Combiner1 : PathCombiner
  TO_INFlow : PMIOPort  Port=1  Side=Right
  TO_OUTFlow : PMIOPort  Port=2  Side=Left
  FROM_INFlow : PMIOPort  Port=3  Side=Right
  FROM_OUTFlow : PMIOPort  Port=4  Side=Left
  wires:
  Get Attribute/2 -> INFlow_Metric/1
  Get Attribute/1 -> OUTFlow_Metric/1
  FlowRecord/1 -> New_FlowRecord/1
  connections:
  Get Attribute/RConn1 -- FIFO Queue/LConn1
  Path Combiner1/RConn1 -- Get Attribute/LConn1
  FROM_OUTFlow/RConn1 -- Path Combiner1/LConn3
  FROM_INFlow/RConn1 -- Path Combiner1/LConn2
  TO_OUTFlow/RConn1 -- Output Switch/RConn2
  TO_INFlow/RConn1 -- Output Switch/RConn1
  Initialize_FlowRecord/RConn1 -- Path Combiner1/LConn1
  New_FlowRecord/RConn1 -- Initialize_FlowRecord/LConn1
  Output Switch/LConn1 -- FIFO Queue/RConn1

== matlab function PickSlowCarton/Calculate_INFlow/Calculate_INFlow ==
  data: UoH input double; INFlow_return output double; Quantity input double; INFlow input double
function INFlow_return  = Calculate_INFlow(UoH, Quantity, INFlow)
%#codegen

INFlow_return = INFlow;


if eq(UoH, 0) == 0
%test if parameters are initialized

    INFlow_return(UoH) = INFlow(UoH) + Quantity;
end

== matlab function PickSlowCarton/Calculate_OUTFlow/Calculate_OUTFlow ==
  data: UoH input double; OUTFlow_return output double; Quantity input double; OUTFlow input double
function OUTFlow_return  = Calculate_OUTFlow(UoH, Quantity, OUTFlow)
%#codegen

OUTFlow_return = OUTFlow;


if eq(UoH, 0) == 0
%test if parameters are initialized

    OUTFlow_return(UoH) = OUTFlow(UoH) + Quantity;
end

== matlab function MixedPallet/Calculate_INFlow/Calculate_INFlow ==
  data: UoH input double; INFlow_return output double; Quantity input double; INFlow input double
function INFlow_return  = Calculate_INFlow(UoH, Quantity, INFlow)
%#codegen

INFlow_return = INFlow;


if eq(UoH, 0) == 0
%test if parameters are initialized

    INFlow_return(UoH) = INFlow(UoH) + Quantity;
end

== matlab function MixedPallet/Calculate_OUTFlow/Calculate_OUTFlow ==
  data: UoH input double; OUTFlow_return output double; Quantity input double; OUTFlow input double
function OUTFlow_return  = Calculate_OUTFlow(UoH, Quantity, OUTFlow)
%#codegen

OUTFlow_return = OUTFlow;


if eq(UoH, 0) == 0
%test if parameters are initialized

    OUTFlow_return(UoH) = OUTFlow(UoH) + Quantity;
end

== matlab function LTL/Calculate_INFlow/Calculate_INFlow ==
  data: UoH input double; INFlow_return output double; Quantity input double; INFlow input double
function INFlow_return  = Calculate_INFlow(UoH, Quantity, INFlow)
%#codegen

INFlow_return = INFlow;


if eq(UoH, 0) == 0
%test if parameters are initialized

    INFlow_return(UoH) = INFlow(UoH) + Quantity;
end

== matlab function HeavyCarton2MPassembly/Calculate_INFlow/Calculate_INFlow ==
  data: UoH input double; INFlow_return output double; Quantity input double; INFlow input double
function INFlow_return  = Calculate_INFlow(UoH, Quantity, INFlow)
%#codegen

INFlow_return = INFlow;


if eq(UoH, 0) == 0
%test if parameters are initialized

    INFlow_return(UoH) = INFlow(UoH) + Quantity;
end

== matlab function HeavyCarton2MPassembly/Calculate_OUTFlow/Calculate_OUTFlow ==
  data: UoH input double; OUTFlow_return output double; Quantity input double; OUTFlow input double
function OUTFlow_return  = Calculate_OUTFlow(UoH, Quantity, OUTFlow)
%#codegen

OUTFlow_return = OUTFlow;


if eq(UoH, 0) == 0
%test if parameters are initialized

    OUTFlow_return(UoH) = OUTFlow(UoH) + Quantity;
end

== matlab function LTL/Calculate_OUTFlow/Calculate_OUTFlow ==
  data: UoH input double; OUTFlow_return output double; Quantity input double; OUTFlow input double
function OUTFlow_return  = Calculate_OUTFlow(UoH, Quantity, OUTFlow)
%#codegen

OUTFlow_return = OUTFlow;


if eq(UoH, 0) == 0
%test if parameters are initialized

    OUTFlow_return(UoH) = OUTFlow(UoH) + Quantity;
end

== matlab function HeavyCartonSTORE/Calculate_INFlow/Calculate_INFlow ==
  data: UoH input double; INFlow_return output double; Quantity input double; INFlow input double
function INFlow_return  = Calculate_INFlow(UoH, Quantity, INFlow)
%#codegen

INFlow_return = INFlow;


if eq(UoH, 0) == 0
%test if parameters are initialized

    INFlow_return(UoH) = INFlow(UoH) + Quantity;
end

== matlab function HeavyCartonSTORE/Calculate_OUTFlow/Calculate_OUTFlow ==
  data: UoH input double; OUTFlow_return output double; Quantity input double; OUTFlow input double
function OUTFlow_return  = Calculate_OUTFlow(UoH, Quantity, OUTFlow)
%#codegen

OUTFlow_return = OUTFlow;


if eq(UoH, 0) == 0
%test if parameters are initialized

    OUTFlow_return(UoH) = OUTFlow(UoH) + Quantity;
end

== matlab function FastCartonSTORE/Calculate_INFlow/Calculate_INFlow ==
  data: UoH input double; INFlow_return output double; Quantity input double; INFlow input double
function INFlow_return  = Calculate_INFlow(UoH, Quantity, INFlow)
%#codegen

INFlow_return = INFlow;


if eq(UoH, 0) == 0
%test if parameters are initialized

    INFlow_return(UoH) = INFlow(UoH) + Quantity;
end

== matlab function FastCartonSTORE/Calculate_OUTFlow/Calculate_OUTFlow ==
  data: UoH input double; OUTFlow_return output double; Quantity input double; OUTFlow input double
function OUTFlow_return  = Calculate_OUTFlow(UoH, Quantity, OUTFlow)
%#codegen

OUTFlow_return = OUTFlow;


if eq(UoH, 0) == 0
%test if parameters are initialized

    OUTFlow_return(UoH) = OUTFlow(UoH) + Quantity;
end

== matlab function SlowCarton2MPassembly/Calculate_INFlow/Calculate_INFlow ==
  data: UoH input double; INFlow_return output double; Quantity input double; INFlow input double
function INFlow_return  = Calculate_INFlow(UoH, Quantity, INFlow)
%#codegen

INFlow_return = INFlow;


if eq(UoH, 0) == 0
%test if parameters are initialized

    INFlow_return(UoH) = INFlow(UoH) + Quantity;
end

== matlab function SlowCarton2MPassembly/Calculate_OUTFlow/Calculate_OUTFlow ==
  data: UoH input double; OUTFlow_return output double; Quantity input double; OUTFlow input double
function OUTFlow_return  = Calculate_OUTFlow(UoH, Quantity, OUTFlow)
%#codegen

OUTFlow_return = OUTFlow;


if eq(UoH, 0) == 0
%test if parameters are initialized

    OUTFlow_return(UoH) = OUTFlow(UoH) + Quantity;
end

== matlab function FastCarton2MPassembly/Calculate_INFlow/Calculate_INFlow ==
  data: UoH input double; INFlow_return output double; Quantity input double; INFlow input double
function INFlow_return  = Calculate_INFlow(UoH, Quantity, INFlow)
%#codegen

INFlow_return = INFlow;


if eq(UoH, 0) == 0
%test if parameters are initialized

    INFlow_return(UoH) = INFlow(UoH) + Quantity;
end

== matlab function FastCarton2MPassembly/Calculate_OUTFlow/Calculate_OUTFlow ==
  data: UoH input double; OUTFlow_return output double; Quantity input double; OUTFlow input double
function OUTFlow_return  = Calculate_OUTFlow(UoH, Quantity, OUTFlow)
%#codegen

OUTFlow_return = OUTFlow;


if eq(UoH, 0) == 0
%test if parameters are initialized

    OUTFlow_return(UoH) = OUTFlow(UoH) + Quantity;
end

== matlab function PickHeavyCarton/Calculate_INFlow/Calculate_INFlow ==
  data: UoH input double; INFlow_return output double; Quantity input double; INFlow input double
function INFlow_return  = Calculate_INFlow(UoH, Quantity, INFlow)
%#codegen

INFlow_return = INFlow;


if eq(UoH, 0) == 0
%test if parameters are initialized

    INFlow_return(UoH) = INFlow(UoH) + Quantity;
end

== matlab function PickHeavyCarton/Calculate_OUTFlow/Calculate_OUTFlow ==
  data: UoH input double; OUTFlow_return output double; Quantity input double; OUTFlow input double
function OUTFlow_return  = Calculate_OUTFlow(UoH, Quantity, OUTFlow)
%#codegen

OUTFlow_return = OUTFlow;


if eq(UoH, 0) == 0
%test if parameters are initialized

    OUTFlow_return(UoH) = OUTFlow(UoH) + Quantity;
end

== matlab function PickFastCarton/Calculate_INFlow/Calculate_INFlow ==
  data: UoH input double; INFlow_return output double; Quantity input double; INFlow input double
function INFlow_return  = Calculate_INFlow(UoH, Quantity, INFlow)
%#codegen

INFlow_return = INFlow;


if eq(UoH, 0) == 0
%test if parameters are initialized

    INFlow_return(UoH) = INFlow(UoH) + Quantity;
end

== matlab function PickFastCarton/Calculate_OUTFlow/Calculate_OUTFlow ==
  data: UoH input double; OUTFlow_return output double; Quantity input double; OUTFlow input double
function OUTFlow_return  = Calculate_OUTFlow(UoH, Quantity, OUTFlow)
%#codegen

OUTFlow_return = OUTFlow;


if eq(UoH, 0) == 0
%test if parameters are initialized

    OUTFlow_return(UoH) = OUTFlow(UoH) + Quantity;
end

== matlab function SlowCartonSTORE/Calculate_INFlow/Calculate_INFlow ==
  data: UoH input double; INFlow_return output double; Quantity input double; INFlow input double
function INFlow_return  = Calculate_INFlow(UoH, Quantity, INFlow)
%#codegen

INFlow_return = INFlow;


if eq(UoH, 0) == 0
%test if parameters are initialized

    INFlow_return(UoH) = INFlow(UoH) + Quantity;
end

== matlab function SlowCartonSTORE/Calculate_OUTFlow/Calculate_OUTFlow ==
  data: UoH input double; OUTFlow_return output double; Quantity input double; OUTFlow input double
function OUTFlow_return  = Calculate_OUTFlow(UoH, Quantity, OUTFlow)
%#codegen

OUTFlow_return = OUTFlow;


if eq(UoH, 0) == 0
%test if parameters are initialized

    OUTFlow_return(UoH) = OUTFlow(UoH) + Quantity;
end
